simulink model "experiment"  (R2020a)
settings: Solver=VariableStepAuto  StartTime=0.0  StopTime=75  RelTol=1e-3
InitFcn:
  | INITexp
values from neighbouring files (symbols this model uses):
  d = 1    [INIT.m]    (also in INITKF.m; INITexp.m; INITnonmpc.m; pendcont.m)
  g = -10    [INIT.m]    (also in INITKF.m; INITexp.m = -9.8; INITnonmpc.m = -9.8; pendcont.m = -9.8)
  K = lqr(A,B,Q,R)    [INIT.m]    (also in INITKF.m; INITexp.m; INITnonmpc.m)
  L = 2    [INIT.m]    (also in INITKF.m; INITexp.m = 0.07; INITnonmpc.m = 0.06; pendcont.m = 0.06)
  M = 5    [INIT.m]    (also in INITKF.m; INITexp.m = 0.32; INITnonmpc.m = 0.08; pendcont.m = 0.08)
  m = 1    [INIT.m]    (also in INITKF.m; INITexp.m = 0.25; INITnonmpc.m = 0.01; pendcont.m = 0.01)
  y0 = [0;0;0.1;0]    [INITexp.m]
settings Model: Creator=Prodigio  LastModifiedBy=Prodigio
settings DataIOCC: ReturnWorkspaceOutputs=off
settings DebuggingCC: ArithmeticOperatorsInVariantConditions=warning
settings SFSimCC: SimUseLocalCustomCode=off  CustomCodeUndefinedFunction=UseInterfaceOnly
settings RTWCC: RTWUseLocalCustomCode=off

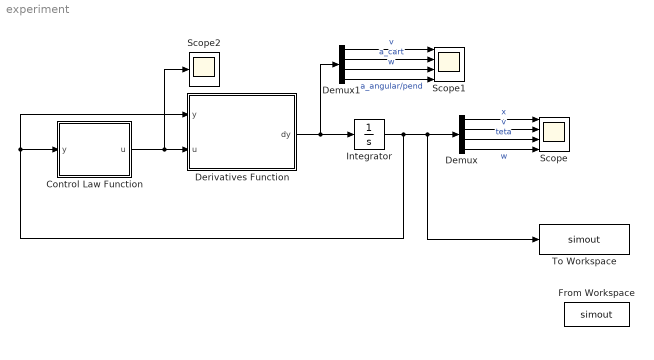
== system experiment ==
  Control Law Function : MATLAB Function  TreatAsAtomicUnit=on
  Demux : Demux
  Demux1 : Demux
  Derivatives Function : MATLAB Function  TreatAsAtomicUnit=on
  From Workspace : FromWorkspace  VariableName=simout
  Integrator : Integrator  InitialCondition=y0
  Scope : Scope  NumInputPorts=4
  Scope1 : Scope  NumInputPorts=4
  Scope2 : Scope
  To Workspace : ToWorkspace  VariableName=simout  SaveFormat=Timeseries  SampleTime=-1
  wires:
  Derivatives Function/1(dy) -> Demux1/1, Integrator/1
  Demux/1 -> Scope/1  "x"
  Demux1/1 -> Scope1/1  "v"
  Demux1/2 -> Scope1/2  "a_cart"
  Control Law Function/1(u) -> Scope2/1, Derivatives Function/2(u)
  Integrator/1 -> Control Law Function/1(y), Derivatives Function/1(y), To Workspace/1, Demux/1
  Demux1/3 -> Scope1/3  "w"
  Demux1/4 -> Scope1/4  "a_angular/pend"
  Demux/3 -> Scope/3  "teta"
  Demux/4 -> Scope/4  "w"
  Demux/2 -> Scope/2  "v"

== matlab function experiment/Control Law Function ==
  data: y input; u output; m parameter; M parameter; L parameter; g parameter; d parameter; K parameter
function u = calc_u_exp(y,m, M, L, g, d, K)
% y = [x , ^x, o , ^o] states , y=xdot
% M massa do carro, m massa do pendulo, L tamanho do fio
% d fricÃ§ao, g grav no pendulo
dy=0*y;
Sy = sin(y(3));
Cy = cos(y(3));
D = m*L*L*(M+m*(1-Cy^2));

% setpoints
% newx = [2; 0; pi; 0];
newx = [0; 0; pi; 0];

% if(t>12)
%     newx = [-1; 0; pi; 0]; 
% end 

% open loop (no control)
% if(t>29)
%   u = 0;
% else
                                            % && u ~= 0
if (( y(3) > (pi-pi/5) ) && ( y(3) < (pi+pi/5)) || ...
   ( y(3) > (-pi-pi/5) ) && ( y(3) < (-pi+pi/5)) )  
    u = K * ([0;0;pi;0] - [y(1);y(2);y(3);y(4)]); % lqr control u = k*(newx-x)
else
    % energy based swing-up control % 1996 furata and astrom eq.6
    % E=2/3*m2*l^2*x(4)^2 - m2*g*l*(cos(x(3))-1);
    % u=0.2*m1*E*x(4)*cos(x(3));
%         k=1;
%         Ed= -m*g*L*cos(pi);
%         E= m*L^2*y(4) - m*g*L*cos(y(3));
%         u=k*y(4)*(E-Ed);
     E= m*g*L*(cos(y(3)));
     u=0.8*M*E*y(4)*(cos(y(3))); %velocidade com que ganha balanço
%     end
end

== matlab function experiment/Derivatives Function ==
  settings: updateMethod=CONTINUOUS
  data: y input; dy output; m parameter; M parameter; L parameter; g parameter; d parameter; K parameter; u input
function dy = derivativesexp(y,m, M, L, g, d, K,u)
% y = [x , ^x, o , ^o] states , y=xdot
% M massa do carro, m massa do pendulo, L tamanho do fio
% d fricÃ§ao, g grav no pendulo
dy=0*y;
Sy = sin(y(3));
Cy = cos(y(3));
D = m*L*L*(M+m*(1-Cy^2));

% setpoints
% newx = [2; 0; pi; 0];
newx = [0; 0; pi; 0];

% if(t>12)
%     newx = [-1; 0; pi; 0]; 
% end 

% open loop (no control)
% if(t>29)
%   u = 0;
% else
                                            % && u ~= 0
if (( y(3) > (pi-pi/5) ) && ( y(3) < (pi+pi/5)) || ...
   ( y(3) > (-pi-pi/5) ) && ( y(3) < (-pi+pi/5)) )  
    u = K * ([0;0;pi;0] - [y(1);y(2);y(3);y(4)]); % lqr control u = k*(newx-x)
else
    % energy based swing-up control % 1996 furata and astrom eq.6
    % E=2/3*m2*l^2*x(4)^2 - m2*g*l*(cos(x(3))-1);
    % u=0.2*m1*E*x(4)*cos(x(3));
%         k=1;
%         Ed= -m*g*L*cos(pi);
%         E= m*L^2*y(4) - m*g*L*cos(y(3));
%         u=k*y(4)*(E-Ed);
     E= m*g*L*(cos(y(3)));
     u=0.8*M*E*y(4)*(cos(y(3))); %velocidade com que ganha balanço
%     end
end



%derivadas 

dy(1,1) = y(2);
dy(2,1) = (1/D)*(-m^2*L^2*g*Cy*Sy + m*L^2*(m*L*y(4)^2*Sy - d*y(2))) + m*L*L*(1/D)*u;
dy(3,1) = y(4);
dy(4,1) = (1/D)*((m+M)*m*g*L*Sy - m*L*Cy*(m*L*y(4)^2*Sy - d*y(2))) - m*L*Cy*(1/D)*u;


% -m*m*l*l*g*Sy*Sy
% m*l*l*m*l*y(4)^2*Sy
% %-m*l*l*d*y(2)
% %m*l*l*u
% 
% (m+M)*m*g*l*Sy
% m*l*Cy*m*l*y(4)^2*Sy
% %-m*l*Cy*d*y(2)
% %m*l*Cy*u
